simulink model "LQRsim_err"  (R2021b)
settings: Solver=VariableStepAuto  StartTime=0.0  StopTime=5  RelTol=1e-3
settings Model: Creator=hty  LastModifiedBy=hty

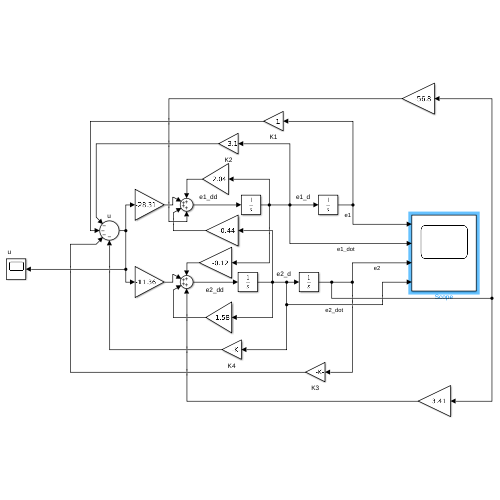
[thumbnail: Simulink's stored preview of the top-level diagram]
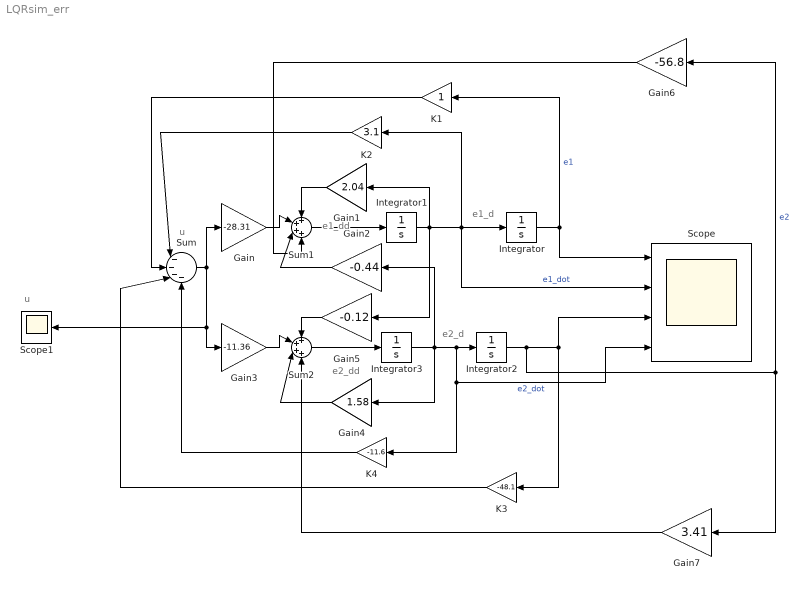
== system LQRsim_err ==
  note: u
  note: u
  note: e2_dd
  note: e2_d
  note: e1_dd
  note: e1_d
  Gain : Gain  Gain=-28.31
  Gain1 : Gain  Gain=2.04
  Gain2 : Gain  Gain=-0.44
  Gain3 : Gain  Gain=-11.36
  Gain4 : Gain  Gain=1.58
  Gain5 : Gain  Gain=-0.12
  Gain6 : Gain  Gain=-56.8
  Gain7 : Gain  Gain=3.41
  Integrator : Integrator  InitialCondition=5
  Integrator1 : Integrator
  Integrator2 : Integrator
  Integrator3 : Integrator
  K1 : Gain
  K2 : Gain  Gain=3.1
  K3 : Gain  Gain=-48.1
  K4 : Gain  Gain=-11.6
  Scope : Scope  NumInputPorts=4
  Scope1 : Scope
  Sum : Sum  Inputs=|----
  Sum1 : Sum  Inputs=++++
  Sum2 : Sum  Inputs=++++
  wires:
  Integrator1/1 -> Gain5/1, Gain1/1, Scope/2, K2/1, Integrator/1  "e1_dot"
  Gain1/1 -> Sum1/1
  Gain3/1 -> Sum2/2
  Sum2/1 -> Integrator3/1
  K3/1 -> Sum/3
  K2/1 -> Sum/1
  Integrator/1 -> K1/1, Scope/1  "e1"
  Gain2/1 -> Sum1/3
  Sum/1 -> Gain3/1, Scope1/1, Gain/1
  Integrator3/1 -> Gain4/1, K4/1, Scope/4, Integrator2/1, Gain2/1  "e2_dot"
  Sum1/1 -> Integrator1/1
  Gain/1 -> Sum1/2
  K1/1 -> Sum/2
  Gain4/1 -> Sum2/3
  K4/1 -> Sum/4
  Integrator2/1 -> Gain7/1, Gain6/1, K3/1, Scope/3  "e2"
  Gain5/1 -> Sum2/1
  Gain7/1 -> Sum2/4
  Gain6/1 -> Sum1/4
